simulink model "project5"  (R2021a)
settings: Solver=VariableStepAuto  StartTime=0.0  StopTime=350  RelTol=1e-3
undefined symbols (not defined in the file or in its folder): AXI4, Lite
libraries: hdlBasic x323, xbsIndex_r4 x1
(part 2 of 3)

== system project5/Subsystem1 ==
  sel_in : Inport
  theta_in : Inport  Port=2
  start : Inport  Port=3
  Data_in2 : Inport  Port=4
  Constant2 : hdlBasic/Constant  const=0  gui_display_data_type=Boolean  arith_type=Boolean  n_bits=16  bin_pt=14  preci_type=Single  exp_width=8  frac_width=24  explicit_period=off  period=1  XmcBlockStatus=1  maskContainerNames=tabcontainer1  block_type=constant  block_config=sysgen:Constant_config
  Constant6 : hdlBasic/Constant  const=0  gui_display_data_type=Fixed-point  arith_type=Signed (2's comp)  n_bits=20  bin_pt=10  preci_type=Single  exp_width=8  frac_width=24  explicit_period=off  period=1  XmcBlockStatus=1  maskContainerNames=tabcontainer1  block_type=constant  block_config=sysgen:Constant_config
  Delay : hdlBasic/Delay  rst=off  en=on  latency=1  reg_retiming=off  XmcBlockStatus=1  maskContainerNames=group1  block_type=delay  block_config=sysgen:Delay_config
  Delay1 : hdlBasic/Delay  rst=off  en=on  latency=1  reg_retiming=off  XmcBlockStatus=1  maskContainerNames=group1  block_type=delay  block_config=sysgen:Delay_config
  Delay2 : hdlBasic/Delay  rst=off  en=off  latency=2  reg_retiming=off  XmcBlockStatus=1  maskContainerNames=group1  block_type=delay  block_config=sysgen:Delay_config
  Delay3 : hdlBasic/Delay  rst=off  en=off  latency=1  reg_retiming=off  XmcBlockStatus=1  maskContainerNames=group1  block_type=delay  block_config=sysgen:Delay_config
  Delay4 : hdlBasic/Delay  rst=off  en=off  latency=1  reg_retiming=off  XmcBlockStatus=1  maskContainerNames=group1  block_type=delay  block_config=sysgen:Delay_config
  Mux : hdlBasic/Mux  inputs=2  en=off  latency=1  precision=Full  arith_type=Unsigned  n_bits=16  bin_pt=14  quantization=Truncate  overflow=Wrap  XmcBlockStatus=1  maskContainerNames=tabcontainer1  block_type=mux  block_config=sysgen:Mux_config
  Mux1 : hdlBasic/Mux  inputs=2  en=off  latency=1  precision=Full  arith_type=Unsigned  n_bits=16  bin_pt=14  quantization=Truncate  overflow=Wrap  XmcBlockStatus=1  maskContainerNames=tabcontainer1  block_type=mux  block_config=sysgen:Mux_config
  Vitis HLS : hdlBasic/Vitis HLS  anytable='C:\ELEC522\jg122\Project5_sinandcos\sincos\solution1'  fast_sim=off  display_datatype=off  rate_propagation_method=Simulink system period  model_file_path=''  latency=1  block_type=vitis_hls
      settings: infoedit=This block allows including C,C++ and SystemC source files in System Generator for DSP designs.
  Ctrl_out : Outport
  theta_out : Outport  Port=2
  result_out : Outport  Port=3
  y_out : Outport  Port=4
  wires:
  Vitis HLS/4 -> Delay/1
  Vitis HLS/5 -> Delay/2
  Delay1/1 -> y_out/1
  Vitis HLS/7 -> Delay1/2
  Vitis HLS/6 -> Delay1/1
  sel_in/1 -> Delay4/1, Mux/1, Mux1/1
  Delay/1 -> result_out/1, Mux/2
  Constant6/1 -> Mux1/3
  Data_in2/1 -> Mux1/2, Mux/3
  Mux1/1 -> Vitis HLS/4
  Mux/1 -> Delay2/1
  theta_in/1 -> Vitis HLS/3, Delay3/1
  Delay3/1 -> theta_out/1
  Delay2/1 -> Vitis HLS/5
  Delay4/1 -> Ctrl_out/1
  start/1 -> Vitis HLS/2
  Constant2/1 -> Vitis HLS/1

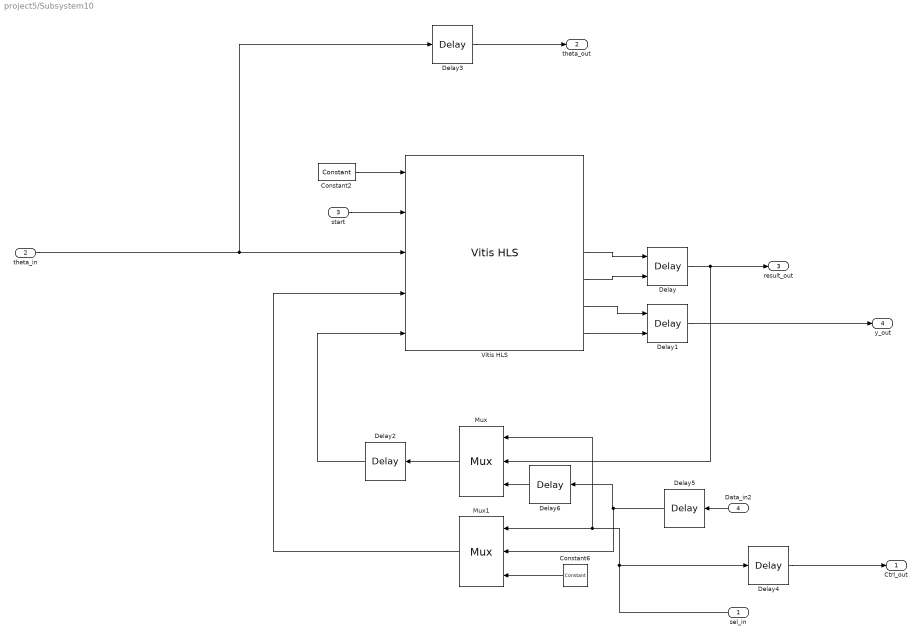
== system project5/Subsystem10 ==
  sel_in : Inport
  theta_in : Inport  Port=2
  start : Inport  Port=3
  Data_in2 : Inport  Port=4
  Constant2 : hdlBasic/Constant  const=0  gui_display_data_type=Boolean  arith_type=Boolean  n_bits=16  bin_pt=14  preci_type=Single  exp_width=8  frac_width=24  explicit_period=off  period=1  XmcBlockStatus=1  maskContainerNames=tabcontainer1  block_type=constant  block_config=sysgen:Constant_config
  Constant6 : hdlBasic/Constant  const=0  gui_display_data_type=Fixed-point  arith_type=Signed (2's comp)  n_bits=20  bin_pt=10  preci_type=Single  exp_width=8  frac_width=24  explicit_period=off  period=1  XmcBlockStatus=1  maskContainerNames=tabcontainer1  block_type=constant  block_config=sysgen:Constant_config
  Delay : hdlBasic/Delay  rst=off  en=on  latency=1  reg_retiming=off  XmcBlockStatus=1  maskContainerNames=group1  block_type=delay  block_config=sysgen:Delay_config
  Delay1 : hdlBasic/Delay  rst=off  en=on  latency=1  reg_retiming=off  XmcBlockStatus=1  maskContainerNames=group1  block_type=delay  block_config=sysgen:Delay_config
  Delay2 : hdlBasic/Delay  rst=off  en=off  latency=2  reg_retiming=off  XmcBlockStatus=1  maskContainerNames=group1  block_type=delay  block_config=sysgen:Delay_config
  Delay3 : hdlBasic/Delay  rst=off  en=off  latency=1  reg_retiming=off  XmcBlockStatus=1  maskContainerNames=group1  block_type=delay  block_config=sysgen:Delay_config
  Delay4 : hdlBasic/Delay  rst=off  en=off  latency=1  reg_retiming=off  XmcBlockStatus=1  maskContainerNames=group1  block_type=delay  block_config=sysgen:Delay_config
  Delay5 : hdlBasic/Delay  rst=off  en=off  latency=19  reg_retiming=off  XmcBlockStatus=1  maskContainerNames=group1  block_type=delay  block_config=sysgen:Delay_config
  Delay6 : hdlBasic/Delay  rst=off  en=off  latency=25  reg_retiming=off  XmcBlockStatus=1  maskContainerNames=group1  block_type=delay  block_config=sysgen:Delay_config
  Mux : hdlBasic/Mux  inputs=2  en=off  latency=1  precision=Full  arith_type=Unsigned  n_bits=16  bin_pt=14  quantization=Truncate  overflow=Wrap  XmcBlockStatus=1  maskContainerNames=tabcontainer1  block_type=mux  block_config=sysgen:Mux_config
  Mux1 : hdlBasic/Mux  inputs=2  en=off  latency=1  precision=Full  arith_type=Unsigned  n_bits=16  bin_pt=14  quantization=Truncate  overflow=Wrap  XmcBlockStatus=1  maskContainerNames=tabcontainer1  block_type=mux  block_config=sysgen:Mux_config
  Vitis HLS : hdlBasic/Vitis HLS  anytable='C:\ELEC522\jg122\Project5_sinandcos\sincos\solution1'  fast_sim=off  display_datatype=off  rate_propagation_method=Simulink system period  model_file_path=''  latency=1  block_type=vitis_hls
      settings: infoedit=This block allows including C,C++ and SystemC source files in System Generator for DSP designs.
  Ctrl_out : Outport
  theta_out : Outport  Port=2
  result_out : Outport  Port=3
  y_out : Outport  Port=4
  wires:
  Vitis HLS/4 -> Delay/1
  Vitis HLS/5 -> Delay/2
  Delay1/1 -> y_out/1
  Vitis HLS/7 -> Delay1/2
  Vitis HLS/6 -> Delay1/1
  Delay/1 -> result_out/1, Mux/2
  Constant6/1 -> Mux1/3
  Data_in2/1 -> Delay5/1
  Mux1/1 -> Vitis HLS/4
  Mux/1 -> Delay2/1
  theta_in/1 -> Vitis HLS/3, Delay3/1
  Delay3/1 -> theta_out/1
  Delay2/1 -> Vitis HLS/5
  Delay4/1 -> Ctrl_out/1
  Delay5/1 -> Mux1/2, Delay6/1
  Delay6/1 -> Mux/3
  sel_in/1 -> Mux/1, Mux1/1, Delay4/1
  start/1 -> Vitis HLS/2
  Constant2/1 -> Vitis HLS/1

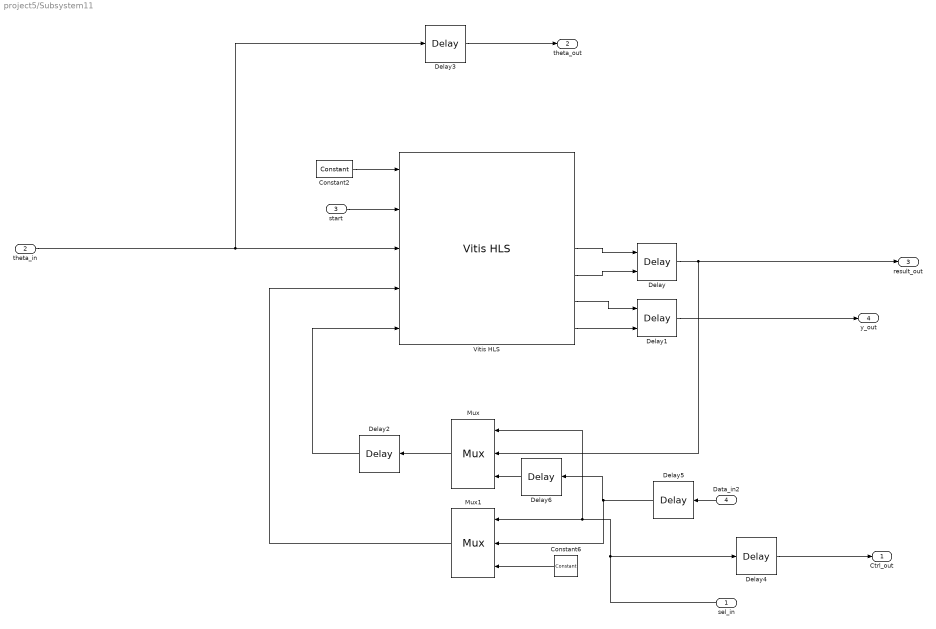
== system project5/Subsystem11 ==
  sel_in : Inport
  theta_in : Inport  Port=2
  start : Inport  Port=3
  Data_in2 : Inport  Port=4
  Constant2 : hdlBasic/Constant  const=0  gui_display_data_type=Boolean  arith_type=Boolean  n_bits=16  bin_pt=14  preci_type=Single  exp_width=8  frac_width=24  explicit_period=off  period=1  XmcBlockStatus=1  maskContainerNames=tabcontainer1  block_type=constant  block_config=sysgen:Constant_config
  Constant6 : hdlBasic/Constant  const=0  gui_display_data_type=Fixed-point  arith_type=Signed (2's comp)  n_bits=20  bin_pt=10  preci_type=Single  exp_width=8  frac_width=24  explicit_period=off  period=1  XmcBlockStatus=1  maskContainerNames=tabcontainer1  block_type=constant  block_config=sysgen:Constant_config
  Delay : hdlBasic/Delay  rst=off  en=on  latency=1  reg_retiming=off  XmcBlockStatus=1  maskContainerNames=group1  block_type=delay  block_config=sysgen:Delay_config
  Delay1 : hdlBasic/Delay  rst=off  en=on  latency=1  reg_retiming=off  XmcBlockStatus=1  maskContainerNames=group1  block_type=delay  block_config=sysgen:Delay_config
  Delay2 : hdlBasic/Delay  rst=off  en=off  latency=2  reg_retiming=off  XmcBlockStatus=1  maskContainerNames=group1  block_type=delay  block_config=sysgen:Delay_config
  Delay3 : hdlBasic/Delay  rst=off  en=off  latency=1  reg_retiming=off  XmcBlockStatus=1  maskContainerNames=group1  block_type=delay  block_config=sysgen:Delay_config
  Delay4 : hdlBasic/Delay  rst=off  en=off  latency=1  reg_retiming=off  XmcBlockStatus=1  maskContainerNames=group1  block_type=delay  block_config=sysgen:Delay_config
  Delay5 : hdlBasic/Delay  rst=off  en=off  latency=19  reg_retiming=off  XmcBlockStatus=1  maskContainerNames=group1  block_type=delay  block_config=sysgen:Delay_config
  Delay6 : hdlBasic/Delay  rst=off  en=off  latency=25  reg_retiming=off  XmcBlockStatus=1  maskContainerNames=group1  block_type=delay  block_config=sysgen:Delay_config
  Mux : hdlBasic/Mux  inputs=2  en=off  latency=1  precision=Full  arith_type=Unsigned  n_bits=16  bin_pt=14  quantization=Truncate  overflow=Wrap  XmcBlockStatus=1  maskContainerNames=tabcontainer1  block_type=mux  block_config=sysgen:Mux_config
  Mux1 : hdlBasic/Mux  inputs=2  en=off  latency=1  precision=Full  arith_type=Unsigned  n_bits=16  bin_pt=14  quantization=Truncate  overflow=Wrap  XmcBlockStatus=1  maskContainerNames=tabcontainer1  block_type=mux  block_config=sysgen:Mux_config
  Vitis HLS : hdlBasic/Vitis HLS  anytable='C:\ELEC522\jg122\Project5_sinandcos\sincos\solution1'  fast_sim=off  display_datatype=off  rate_propagation_method=Simulink system period  model_file_path=''  latency=1  block_type=vitis_hls
      settings: infoedit=This block allows including C,C++ and SystemC source files in System Generator for DSP designs.
  Ctrl_out : Outport
  theta_out : Outport  Port=2
  result_out : Outport  Port=3
  y_out : Outport  Port=4
  wires:
  Vitis HLS/4 -> Delay/1
  Vitis HLS/5 -> Delay/2
  Delay1/1 -> y_out/1
  Vitis HLS/7 -> Delay1/2
  Vitis HLS/6 -> Delay1/1
  Constant6/1 -> Mux1/3
  Data_in2/1 -> Delay5/1
  Mux1/1 -> Vitis HLS/4
  Mux/1 -> Delay2/1
  theta_in/1 -> Vitis HLS/3, Delay3/1
  Delay3/1 -> theta_out/1
  Delay2/1 -> Vitis HLS/5
  Delay4/1 -> Ctrl_out/1
  Delay5/1 -> Mux1/2, Delay6/1
  Delay6/1 -> Mux/3
  sel_in/1 -> Mux/1, Mux1/1, Delay4/1
  start/1 -> Vitis HLS/2
  Constant2/1 -> Vitis HLS/1
  Delay/1 -> result_out/1, Mux/2

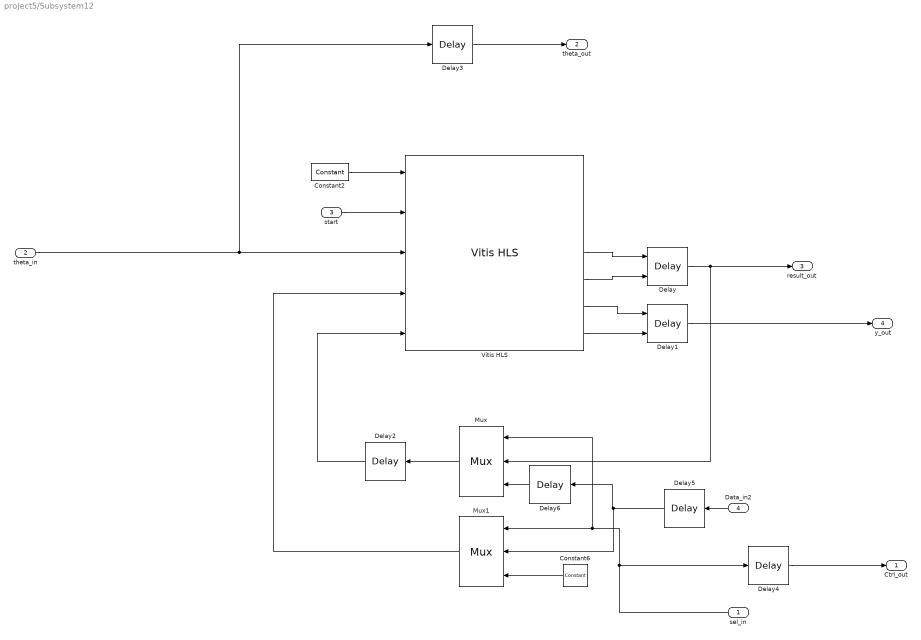
== system project5/Subsystem12 ==
  sel_in : Inport
  theta_in : Inport  Port=2
  start : Inport  Port=3
  Data_in2 : Inport  Port=4
  Constant2 : hdlBasic/Constant  const=0  gui_display_data_type=Boolean  arith_type=Boolean  n_bits=16  bin_pt=14  preci_type=Single  exp_width=8  frac_width=24  explicit_period=off  period=1  XmcBlockStatus=1  maskContainerNames=tabcontainer1  block_type=constant  block_config=sysgen:Constant_config
  Constant6 : hdlBasic/Constant  const=0  gui_display_data_type=Fixed-point  arith_type=Signed (2's comp)  n_bits=20  bin_pt=10  preci_type=Single  exp_width=8  frac_width=24  explicit_period=off  period=1  XmcBlockStatus=1  maskContainerNames=tabcontainer1  block_type=constant  block_config=sysgen:Constant_config
  Delay : hdlBasic/Delay  rst=off  en=on  latency=1  reg_retiming=off  XmcBlockStatus=1  maskContainerNames=group1  block_type=delay  block_config=sysgen:Delay_config
  Delay1 : hdlBasic/Delay  rst=off  en=on  latency=1  reg_retiming=off  XmcBlockStatus=1  maskContainerNames=group1  block_type=delay  block_config=sysgen:Delay_config
  Delay2 : hdlBasic/Delay  rst=off  en=off  latency=2  reg_retiming=off  XmcBlockStatus=1  maskContainerNames=group1  block_type=delay  block_config=sysgen:Delay_config
  Delay3 : hdlBasic/Delay  rst=off  en=off  latency=1  reg_retiming=off  XmcBlockStatus=1  maskContainerNames=group1  block_type=delay  block_config=sysgen:Delay_config
  Delay4 : hdlBasic/Delay  rst=off  en=off  latency=1  reg_retiming=off  XmcBlockStatus=1  maskContainerNames=group1  block_type=delay  block_config=sysgen:Delay_config
  Delay5 : hdlBasic/Delay  rst=off  en=off  latency=19  reg_retiming=off  XmcBlockStatus=1  maskContainerNames=group1  block_type=delay  block_config=sysgen:Delay_config
  Delay6 : hdlBasic/Delay  rst=off  en=off  latency=25  reg_retiming=off  XmcBlockStatus=1  maskContainerNames=group1  block_type=delay  block_config=sysgen:Delay_config
  Mux : hdlBasic/Mux  inputs=2  en=off  latency=1  precision=Full  arith_type=Unsigned  n_bits=16  bin_pt=14  quantization=Truncate  overflow=Wrap  XmcBlockStatus=1  maskContainerNames=tabcontainer1  block_type=mux  block_config=sysgen:Mux_config
  Mux1 : hdlBasic/Mux  inputs=2  en=off  latency=1  precision=Full  arith_type=Unsigned  n_bits=16  bin_pt=14  quantization=Truncate  overflow=Wrap  XmcBlockStatus=1  maskContainerNames=tabcontainer1  block_type=mux  block_config=sysgen:Mux_config
  Vitis HLS : hdlBasic/Vitis HLS  anytable='C:\ELEC522\jg122\Project5_sinandcos\sincos\solution1'  fast_sim=off  display_datatype=off  rate_propagation_method=Simulink system period  model_file_path=''  latency=1  block_type=vitis_hls
      settings: infoedit=This block allows including C,C++ and SystemC source files in System Generator for DSP designs.
  Ctrl_out : Outport
  theta_out : Outport  Port=2
  result_out : Outport  Port=3
  y_out : Outport  Port=4
  wires:
  Vitis HLS/4 -> Delay/1
  Vitis HLS/5 -> Delay/2
  Delay1/1 -> y_out/1
  Vitis HLS/7 -> Delay1/2
  Vitis HLS/6 -> Delay1/1
  Constant6/1 -> Mux1/3
  Data_in2/1 -> Delay5/1
  Mux1/1 -> Vitis HLS/4
  Mux/1 -> Delay2/1
  theta_in/1 -> Vitis HLS/3, Delay3/1
  Delay3/1 -> theta_out/1
  Delay2/1 -> Vitis HLS/5
  Delay4/1 -> Ctrl_out/1
  Delay5/1 -> Mux1/2, Delay6/1
  Delay6/1 -> Mux/3
  sel_in/1 -> Mux/1, Mux1/1, Delay4/1
  start/1 -> Vitis HLS/2
  Constant2/1 -> Vitis HLS/1
  Delay/1 -> result_out/1, Mux/2

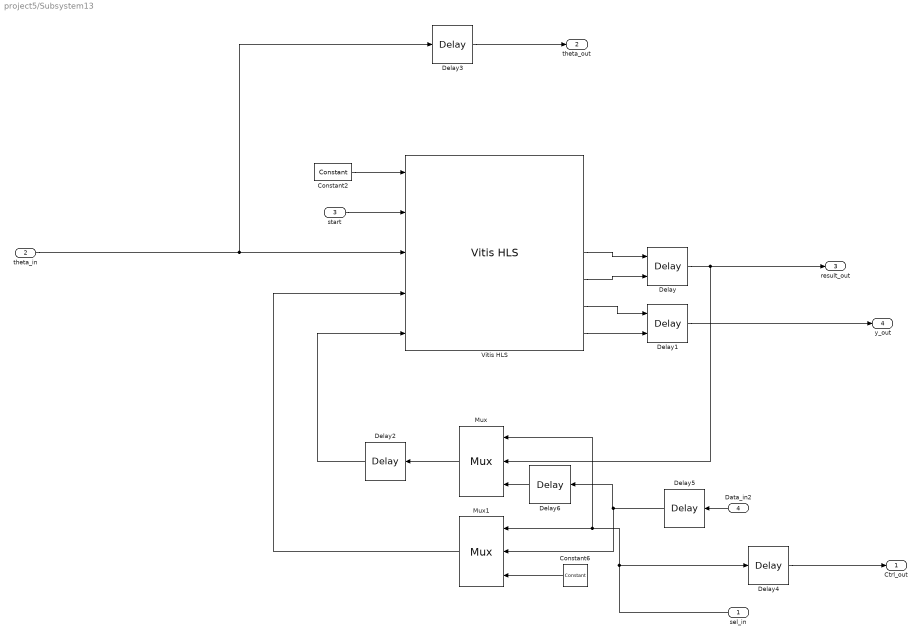
== system project5/Subsystem13 ==
  sel_in : Inport
  theta_in : Inport  Port=2
  start : Inport  Port=3
  Data_in2 : Inport  Port=4
  Constant2 : hdlBasic/Constant  const=0  gui_display_data_type=Boolean  arith_type=Boolean  n_bits=16  bin_pt=14  preci_type=Single  exp_width=8  frac_width=24  explicit_period=off  period=1  XmcBlockStatus=1  maskContainerNames=tabcontainer1  block_type=constant  block_config=sysgen:Constant_config
  Constant6 : hdlBasic/Constant  const=0  gui_display_data_type=Fixed-point  arith_type=Signed (2's comp)  n_bits=20  bin_pt=10  preci_type=Single  exp_width=8  frac_width=24  explicit_period=off  period=1  XmcBlockStatus=1  maskContainerNames=tabcontainer1  block_type=constant  block_config=sysgen:Constant_config
  Delay : hdlBasic/Delay  rst=off  en=on  latency=1  reg_retiming=off  XmcBlockStatus=1  maskContainerNames=group1  block_type=delay  block_config=sysgen:Delay_config
  Delay1 : hdlBasic/Delay  rst=off  en=on  latency=1  reg_retiming=off  XmcBlockStatus=1  maskContainerNames=group1  block_type=delay  block_config=sysgen:Delay_config
  Delay2 : hdlBasic/Delay  rst=off  en=off  latency=2  reg_retiming=off  XmcBlockStatus=1  maskContainerNames=group1  block_type=delay  block_config=sysgen:Delay_config
  Delay3 : hdlBasic/Delay  rst=off  en=off  latency=1  reg_retiming=off  XmcBlockStatus=1  maskContainerNames=group1  block_type=delay  block_config=sysgen:Delay_config
  Delay4 : hdlBasic/Delay  rst=off  en=off  latency=1  reg_retiming=off  XmcBlockStatus=1  maskContainerNames=group1  block_type=delay  block_config=sysgen:Delay_config
  Delay5 : hdlBasic/Delay  rst=off  en=off  latency=19  reg_retiming=off  XmcBlockStatus=1  maskContainerNames=group1  block_type=delay  block_config=sysgen:Delay_config
  Delay6 : hdlBasic/Delay  rst=off  en=off  latency=25  reg_retiming=off  XmcBlockStatus=1  maskContainerNames=group1  block_type=delay  block_config=sysgen:Delay_config
  Mux : hdlBasic/Mux  inputs=2  en=off  latency=1  precision=Full  arith_type=Unsigned  n_bits=16  bin_pt=14  quantization=Truncate  overflow=Wrap  XmcBlockStatus=1  maskContainerNames=tabcontainer1  block_type=mux  block_config=sysgen:Mux_config
  Mux1 : hdlBasic/Mux  inputs=2  en=off  latency=1  precision=Full  arith_type=Unsigned  n_bits=16  bin_pt=14  quantization=Truncate  overflow=Wrap  XmcBlockStatus=1  maskContainerNames=tabcontainer1  block_type=mux  block_config=sysgen:Mux_config
  Vitis HLS : hdlBasic/Vitis HLS  anytable='C:\ELEC522\jg122\Project5_sinandcos\sincos\solution1'  fast_sim=off  display_datatype=off  rate_propagation_method=Simulink system period  model_file_path=''  latency=1  block_type=vitis_hls
      settings: infoedit=This block allows including C,C++ and SystemC source files in System Generator for DSP designs.
  Ctrl_out : Outport
  theta_out : Outport  Port=2
  result_out : Outport  Port=3
  y_out : Outport  Port=4
  wires:
  Vitis HLS/4 -> Delay/1
  Vitis HLS/5 -> Delay/2
  Delay1/1 -> y_out/1
  Vitis HLS/7 -> Delay1/2
  Vitis HLS/6 -> Delay1/1
  Constant6/1 -> Mux1/3
  Data_in2/1 -> Delay5/1
  Mux1/1 -> Vitis HLS/4
  Mux/1 -> Delay2/1
  theta_in/1 -> Vitis HLS/3, Delay3/1
  Delay3/1 -> theta_out/1
  Delay2/1 -> Vitis HLS/5
  Delay4/1 -> Ctrl_out/1
  Delay5/1 -> Mux1/2, Delay6/1
  Delay6/1 -> Mux/3
  sel_in/1 -> Mux/1, Mux1/1, Delay4/1
  start/1 -> Vitis HLS/2
  Constant2/1 -> Vitis HLS/1
  Delay/1 -> result_out/1, Mux/2

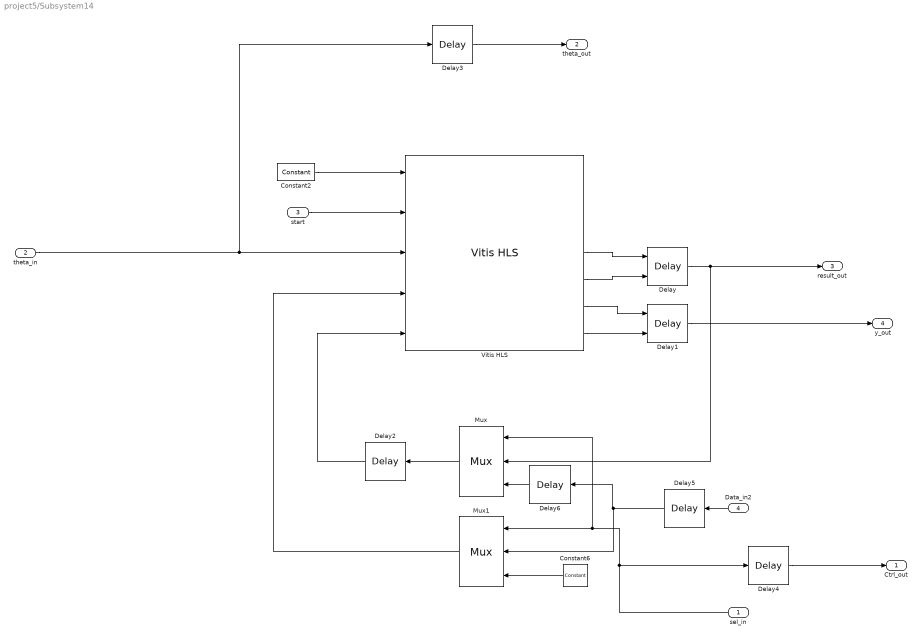
== system project5/Subsystem14 ==
  sel_in : Inport
  theta_in : Inport  Port=2
  start : Inport  Port=3
  Data_in2 : Inport  Port=4
  Constant2 : hdlBasic/Constant  const=0  gui_display_data_type=Boolean  arith_type=Boolean  n_bits=16  bin_pt=14  preci_type=Single  exp_width=8  frac_width=24  explicit_period=off  period=1  XmcBlockStatus=1  maskContainerNames=tabcontainer1  block_type=constant  block_config=sysgen:Constant_config
  Constant6 : hdlBasic/Constant  const=0  gui_display_data_type=Fixed-point  arith_type=Signed (2's comp)  n_bits=20  bin_pt=10  preci_type=Single  exp_width=8  frac_width=24  explicit_period=off  period=1  XmcBlockStatus=1  maskContainerNames=tabcontainer1  block_type=constant  block_config=sysgen:Constant_config
  Delay : hdlBasic/Delay  rst=off  en=on  latency=1  reg_retiming=off  XmcBlockStatus=1  maskContainerNames=group1  block_type=delay  block_config=sysgen:Delay_config
  Delay1 : hdlBasic/Delay  rst=off  en=on  latency=1  reg_retiming=off  XmcBlockStatus=1  maskContainerNames=group1  block_type=delay  block_config=sysgen:Delay_config
  Delay2 : hdlBasic/Delay  rst=off  en=off  latency=2  reg_retiming=off  XmcBlockStatus=1  maskContainerNames=group1  block_type=delay  block_config=sysgen:Delay_config
  Delay3 : hdlBasic/Delay  rst=off  en=off  latency=1  reg_retiming=off  XmcBlockStatus=1  maskContainerNames=group1  block_type=delay  block_config=sysgen:Delay_config
  Delay4 : hdlBasic/Delay  rst=off  en=off  latency=1  reg_retiming=off  XmcBlockStatus=1  maskContainerNames=group1  block_type=delay  block_config=sysgen:Delay_config
  Delay5 : hdlBasic/Delay  rst=off  en=off  latency=19  reg_retiming=off  XmcBlockStatus=1  maskContainerNames=group1  block_type=delay  block_config=sysgen:Delay_config
  Delay6 : hdlBasic/Delay  rst=off  en=off  latency=25  reg_retiming=off  XmcBlockStatus=1  maskContainerNames=group1  block_type=delay  block_config=sysgen:Delay_config
  Mux : hdlBasic/Mux  inputs=2  en=off  latency=1  precision=Full  arith_type=Unsigned  n_bits=16  bin_pt=14  quantization=Truncate  overflow=Wrap  XmcBlockStatus=1  maskContainerNames=tabcontainer1  block_type=mux  block_config=sysgen:Mux_config
  Mux1 : hdlBasic/Mux  inputs=2  en=off  latency=1  precision=Full  arith_type=Unsigned  n_bits=16  bin_pt=14  quantization=Truncate  overflow=Wrap  XmcBlockStatus=1  maskContainerNames=tabcontainer1  block_type=mux  block_config=sysgen:Mux_config
  Vitis HLS : hdlBasic/Vitis HLS  anytable='C:\ELEC522\jg122\Project5_sinandcos\sincos\solution1'  fast_sim=off  display_datatype=off  rate_propagation_method=Simulink system period  model_file_path=''  latency=1  block_type=vitis_hls
      settings: infoedit=This block allows including C,C++ and SystemC source files in System Generator for DSP designs.
  Ctrl_out : Outport
  theta_out : Outport  Port=2
  result_out : Outport  Port=3
  y_out : Outport  Port=4
  wires:
  Vitis HLS/4 -> Delay/1
  Vitis HLS/5 -> Delay/2
  Delay1/1 -> y_out/1
  Vitis HLS/7 -> Delay1/2
  Vitis HLS/6 -> Delay1/1
  Constant6/1 -> Mux1/3
  Data_in2/1 -> Delay5/1
  Mux1/1 -> Vitis HLS/4
  Mux/1 -> Delay2/1
  theta_in/1 -> Vitis HLS/3, Delay3/1
  Delay3/1 -> theta_out/1
  Delay2/1 -> Vitis HLS/5
  Delay4/1 -> Ctrl_out/1
  Delay5/1 -> Mux1/2, Delay6/1
  Delay6/1 -> Mux/3
  sel_in/1 -> Mux/1, Mux1/1, Delay4/1
  start/1 -> Vitis HLS/2
  Constant2/1 -> Vitis HLS/1
  Delay/1 -> result_out/1, Mux/2

== system project5/Subsystem15 ==
  SIgnal_ctrl : Inport
  Signal_input1 : Inport  Port=2
  start : Inport  Port=3
  Constant1 : hdlBasic/Constant  const=0  gui_display_data_type=Boolean  arith_type=Boolean  n_bits=16  bin_pt=14  preci_type=Single  exp_width=8  frac_width=24  explicit_period=off  period=1  XmcBlockStatus=1  maskContainerNames=tabcontainer1  block_type=constant  block_config=sysgen:Constant_config
  Constant3 : hdlBasic/Constant  const=0  gui_display_data_type=Fixed-point  arith_type=Signed (2's comp)  n_bits=20  bin_pt=10  preci_type=Single  exp_width=8  frac_width=24  explicit_period=off  period=1  XmcBlockStatus=1  maskContainerNames=tabcontainer1  block_type=constant  block_config=sysgen:Constant_config
  Delay1 : hdlBasic/Delay  rst=off  en=off  latency=5  reg_retiming=off  XmcBlockStatus=1  maskContainerNames=group1  block_type=delay  block_config=sysgen:Delay_config
  Delay2 : hdlBasic/Delay  rst=off  en=off  latency=2  reg_retiming=off  XmcBlockStatus=1  maskContainerNames=group1  block_type=delay  block_config=sysgen:Delay_config
  Delay3 : hdlBasic/Delay  rst=off  en=off  latency=20  reg_retiming=off  XmcBlockStatus=1  maskContainerNames=group1  block_type=delay  block_config=sysgen:Delay_config
  Delay4 : hdlBasic/Delay  rst=off  en=on  latency=1  reg_retiming=off  XmcBlockStatus=1  maskContainerNames=group1  block_type=delay  block_config=sysgen:Delay_config
  Delay5 : hdlBasic/Delay  rst=off  en=on  latency=1  reg_retiming=off  XmcBlockStatus=1  maskContainerNames=group1  block_type=delay  block_config=sysgen:Delay_config
  Delay6 : hdlBasic/Delay  rst=off  en=off  latency=25  reg_retiming=off  XmcBlockStatus=1  maskContainerNames=group1  block_type=delay  block_config=sysgen:Delay_config
  Delay7 : hdlBasic/Delay  rst=off  en=off  latency=79  reg_retiming=off  XmcBlockStatus=1  maskContainerNames=group1  block_type=delay  block_config=sysgen:Delay_config
  Delay8 : hdlBasic/Delay  rst=off  en=off  latency=23  reg_retiming=off  XmcBlockStatus=1  maskContainerNames=group1  block_type=delay  block_config=sysgen:Delay_config
  Mux : hdlBasic/Mux  inputs=2  en=off  latency=1  precision=Full  arith_type=Unsigned  n_bits=16  bin_pt=14  quantization=Truncate  overflow=Wrap  XmcBlockStatus=1  maskContainerNames=tabcontainer1  block_type=mux  block_config=sysgen:Mux_config
  Mux1 : hdlBasic/Mux  inputs=2  en=off  latency=1  precision=Full  arith_type=Unsigned  n_bits=16  bin_pt=14  quantization=Truncate  overflow=Wrap  XmcBlockStatus=1  maskContainerNames=tabcontainer1  block_type=mux  block_config=sysgen:Mux_config
  Vitis HLS : hdlBasic/Vitis HLS  anytable='C:\ELEC522\jg122\Project5_atan\atan\solution1'  fast_sim=off  display_datatype=on  rate_propagation_method=Simulink system period  model_file_path=''  latency=1  block_type=vitis_hls
      settings: infoedit=This block allows including C,C++ and SystemC source files in System Generator for DSP designs.
  Ctrl_out : Outport
  atan_out1 : Outport  Port=2
  R_out : Outport  Port=3
  wires:
  Vitis HLS/4 -> Delay4/1
  Vitis HLS/6 -> Delay5/1, Delay1/1
  SIgnal_ctrl/1 -> Delay7/1
  Constant3/1 -> Mux1/3
  Mux/1 -> Delay2/1
  Vitis HLS/5 -> Delay4/2
  Vitis HLS/7 -> Delay5/2
  Delay4/1 -> atan_out1/1
  Delay2/1 -> Vitis HLS/3
  Mux1/1 -> Vitis HLS/4
  Delay5/1 -> Delay8/1
  Delay3/1 -> Ctrl_out/1
  Delay1/1 -> Mux/2
  Delay7/1 -> Mux1/1, Delay3/1, Mux/1
  Signal_input1/1 -> Delay6/1, Mux1/2
  Delay6/1 -> Mux/3
  Delay8/1 -> R_out/1
  start/1 -> Vitis HLS/2
  Constant1/1 -> Vitis HLS/1

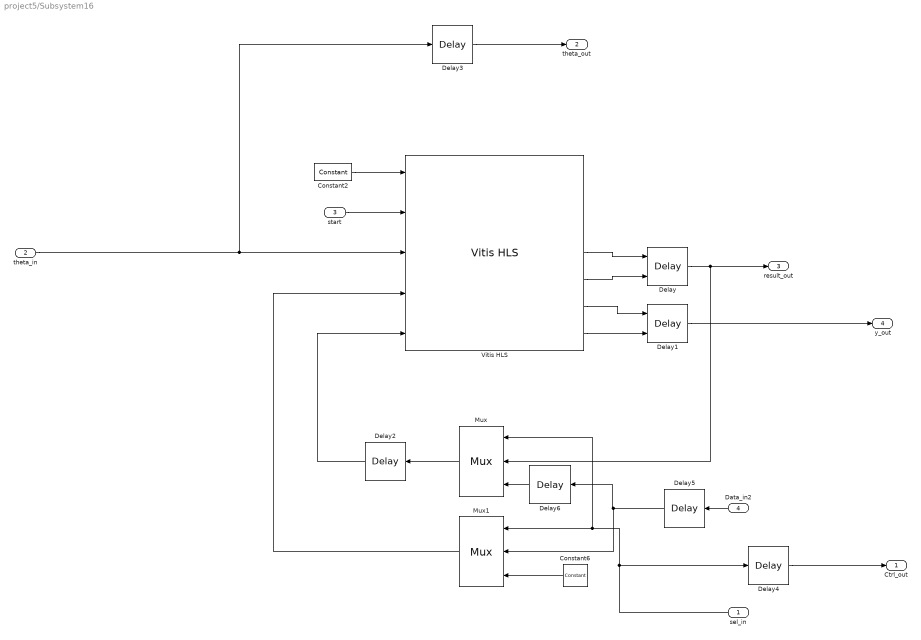
== system project5/Subsystem16 ==
  sel_in : Inport
  theta_in : Inport  Port=2
  start : Inport  Port=3
  Data_in2 : Inport  Port=4
  Constant2 : hdlBasic/Constant  const=0  gui_display_data_type=Boolean  arith_type=Boolean  n_bits=16  bin_pt=14  preci_type=Single  exp_width=8  frac_width=24  explicit_period=off  period=1  XmcBlockStatus=1  maskContainerNames=tabcontainer1  block_type=constant  block_config=sysgen:Constant_config
  Constant6 : hdlBasic/Constant  const=0  gui_display_data_type=Fixed-point  arith_type=Signed (2's comp)  n_bits=20  bin_pt=10  preci_type=Single  exp_width=8  frac_width=24  explicit_period=off  period=1  XmcBlockStatus=1  maskContainerNames=tabcontainer1  block_type=constant  block_config=sysgen:Constant_config
  Delay : hdlBasic/Delay  rst=off  en=on  latency=1  reg_retiming=off  XmcBlockStatus=1  maskContainerNames=group1  block_type=delay  block_config=sysgen:Delay_config
  Delay1 : hdlBasic/Delay  rst=off  en=on  latency=1  reg_retiming=off  XmcBlockStatus=1  maskContainerNames=group1  block_type=delay  block_config=sysgen:Delay_config
  Delay2 : hdlBasic/Delay  rst=off  en=off  latency=2  reg_retiming=off  XmcBlockStatus=1  maskContainerNames=group1  block_type=delay  block_config=sysgen:Delay_config
  Delay3 : hdlBasic/Delay  rst=off  en=off  latency=1  reg_retiming=off  XmcBlockStatus=1  maskContainerNames=group1  block_type=delay  block_config=sysgen:Delay_config
  Delay4 : hdlBasic/Delay  rst=off  en=off  latency=1  reg_retiming=off  XmcBlockStatus=1  maskContainerNames=group1  block_type=delay  block_config=sysgen:Delay_config
  Delay5 : hdlBasic/Delay  rst=off  en=off  latency=19  reg_retiming=off  XmcBlockStatus=1  maskContainerNames=group1  block_type=delay  block_config=sysgen:Delay_config
  Delay6 : hdlBasic/Delay  rst=off  en=off  latency=25  reg_retiming=off  XmcBlockStatus=1  maskContainerNames=group1  block_type=delay  block_config=sysgen:Delay_config
  Mux : hdlBasic/Mux  inputs=2  en=off  latency=1  precision=Full  arith_type=Unsigned  n_bits=16  bin_pt=14  quantization=Truncate  overflow=Wrap  XmcBlockStatus=1  maskContainerNames=tabcontainer1  block_type=mux  block_config=sysgen:Mux_config
  Mux1 : hdlBasic/Mux  inputs=2  en=off  latency=1  precision=Full  arith_type=Unsigned  n_bits=16  bin_pt=14  quantization=Truncate  overflow=Wrap  XmcBlockStatus=1  maskContainerNames=tabcontainer1  block_type=mux  block_config=sysgen:Mux_config
  Vitis HLS : hdlBasic/Vitis HLS  anytable='C:\ELEC522\jg122\Project5_sinandcos\sincos\solution1'  fast_sim=off  display_datatype=off  rate_propagation_method=Simulink system period  model_file_path=''  latency=1  block_type=vitis_hls
      settings: infoedit=This block allows including C,C++ and SystemC source files in System Generator for DSP designs.
  Ctrl_out : Outport
  theta_out : Outport  Port=2
  result_out : Outport  Port=3
  y_out : Outport  Port=4
  wires:
  Vitis HLS/4 -> Delay/1
  Vitis HLS/5 -> Delay/2
  Delay1/1 -> y_out/1
  Vitis HLS/7 -> Delay1/2
  Vitis HLS/6 -> Delay1/1
  Delay/1 -> result_out/1, Mux/2
  Constant6/1 -> Mux1/3
  Data_in2/1 -> Delay5/1
  Mux1/1 -> Vitis HLS/4
  Mux/1 -> Delay2/1
  theta_in/1 -> Vitis HLS/3, Delay3/1
  Delay3/1 -> theta_out/1
  Delay2/1 -> Vitis HLS/5
  Delay4/1 -> Ctrl_out/1
  Delay5/1 -> Mux1/2, Delay6/1
  Delay6/1 -> Mux/3
  sel_in/1 -> Mux/1, Mux1/1, Delay4/1
  start/1 -> Vitis HLS/2
  Constant2/1 -> Vitis HLS/1

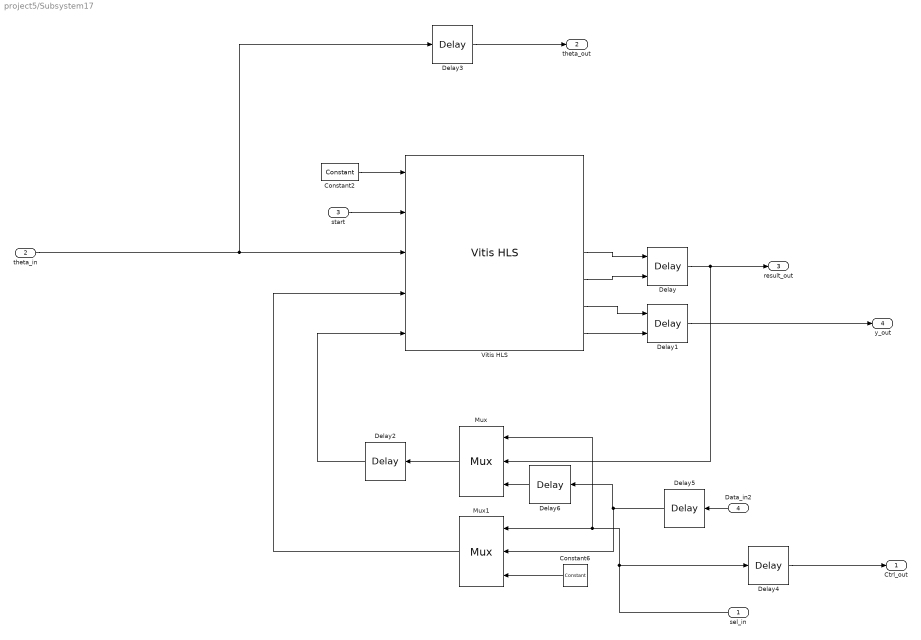
== system project5/Subsystem17 ==
  sel_in : Inport
  theta_in : Inport  Port=2
  start : Inport  Port=3
  Data_in2 : Inport  Port=4
  Constant2 : hdlBasic/Constant  const=0  gui_display_data_type=Boolean  arith_type=Boolean  n_bits=16  bin_pt=14  preci_type=Single  exp_width=8  frac_width=24  explicit_period=off  period=1  XmcBlockStatus=1  maskContainerNames=tabcontainer1  block_type=constant  block_config=sysgen:Constant_config
  Constant6 : hdlBasic/Constant  const=0  gui_display_data_type=Fixed-point  arith_type=Signed (2's comp)  n_bits=20  bin_pt=10  preci_type=Single  exp_width=8  frac_width=24  explicit_period=off  period=1  XmcBlockStatus=1  maskContainerNames=tabcontainer1  block_type=constant  block_config=sysgen:Constant_config
  Delay : hdlBasic/Delay  rst=off  en=on  latency=1  reg_retiming=off  XmcBlockStatus=1  maskContainerNames=group1  block_type=delay  block_config=sysgen:Delay_config
  Delay1 : hdlBasic/Delay  rst=off  en=on  latency=1  reg_retiming=off  XmcBlockStatus=1  maskContainerNames=group1  block_type=delay  block_config=sysgen:Delay_config
  Delay2 : hdlBasic/Delay  rst=off  en=off  latency=2  reg_retiming=off  XmcBlockStatus=1  maskContainerNames=group1  block_type=delay  block_config=sysgen:Delay_config
  Delay3 : hdlBasic/Delay  rst=off  en=off  latency=1  reg_retiming=off  XmcBlockStatus=1  maskContainerNames=group1  block_type=delay  block_config=sysgen:Delay_config
  Delay4 : hdlBasic/Delay  rst=off  en=off  latency=1  reg_retiming=off  XmcBlockStatus=1  maskContainerNames=group1  block_type=delay  block_config=sysgen:Delay_config
  Delay5 : hdlBasic/Delay  rst=off  en=off  latency=19  reg_retiming=off  XmcBlockStatus=1  maskContainerNames=group1  block_type=delay  block_config=sysgen:Delay_config
  Delay6 : hdlBasic/Delay  rst=off  en=off  latency=25  reg_retiming=off  XmcBlockStatus=1  maskContainerNames=group1  block_type=delay  block_config=sysgen:Delay_config
  Mux : hdlBasic/Mux  inputs=2  en=off  latency=1  precision=Full  arith_type=Unsigned  n_bits=16  bin_pt=14  quantization=Truncate  overflow=Wrap  XmcBlockStatus=1  maskContainerNames=tabcontainer1  block_type=mux  block_config=sysgen:Mux_config
  Mux1 : hdlBasic/Mux  inputs=2  en=off  latency=1  precision=Full  arith_type=Unsigned  n_bits=16  bin_pt=14  quantization=Truncate  overflow=Wrap  XmcBlockStatus=1  maskContainerNames=tabcontainer1  block_type=mux  block_config=sysgen:Mux_config
  Vitis HLS : hdlBasic/Vitis HLS  anytable='C:\ELEC522\jg122\Project5_sinandcos\sincos\solution1'  fast_sim=off  display_datatype=off  rate_propagation_method=Simulink system period  model_file_path=''  latency=1  block_type=vitis_hls
      settings: infoedit=This block allows including C,C++ and SystemC source files in System Generator for DSP designs.
  Ctrl_out : Outport
  theta_out : Outport  Port=2
  result_out : Outport  Port=3
  y_out : Outport  Port=4
  wires:
  Vitis HLS/4 -> Delay/1
  Vitis HLS/5 -> Delay/2
  Delay1/1 -> y_out/1
  Vitis HLS/7 -> Delay1/2
  Vitis HLS/6 -> Delay1/1
  Delay/1 -> result_out/1, Mux/2
  Constant6/1 -> Mux1/3
  Data_in2/1 -> Delay5/1
  Mux1/1 -> Vitis HLS/4
  Mux/1 -> Delay2/1
  theta_in/1 -> Vitis HLS/3, Delay3/1
  Delay3/1 -> theta_out/1
  Delay2/1 -> Vitis HLS/5
  Delay4/1 -> Ctrl_out/1
  Delay5/1 -> Mux1/2, Delay6/1
  Delay6/1 -> Mux/3
  sel_in/1 -> Mux/1, Mux1/1, Delay4/1
  Constant2/1 -> Vitis HLS/1
  start/1 -> Vitis HLS/2

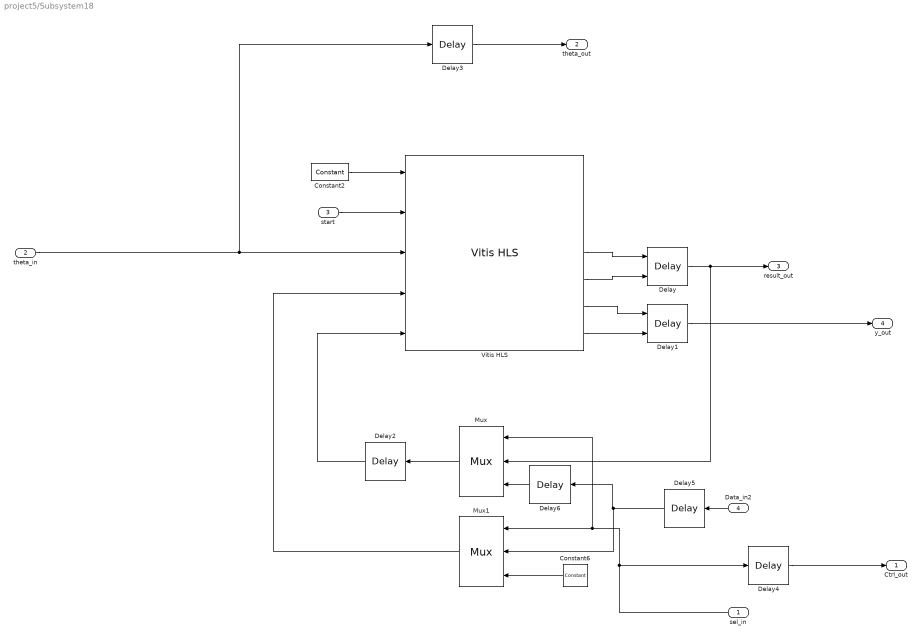
== system project5/Subsystem18 ==
  sel_in : Inport
  theta_in : Inport  Port=2
  start : Inport  Port=3
  Data_in2 : Inport  Port=4
  Constant2 : hdlBasic/Constant  const=0  gui_display_data_type=Boolean  arith_type=Boolean  n_bits=16  bin_pt=14  preci_type=Single  exp_width=8  frac_width=24  explicit_period=off  period=1  XmcBlockStatus=1  maskContainerNames=tabcontainer1  block_type=constant  block_config=sysgen:Constant_config
  Constant6 : hdlBasic/Constant  const=0  gui_display_data_type=Fixed-point  arith_type=Signed (2's comp)  n_bits=20  bin_pt=10  preci_type=Single  exp_width=8  frac_width=24  explicit_period=off  period=1  XmcBlockStatus=1  maskContainerNames=tabcontainer1  block_type=constant  block_config=sysgen:Constant_config
  Delay : hdlBasic/Delay  rst=off  en=on  latency=1  reg_retiming=off  XmcBlockStatus=1  maskContainerNames=group1  block_type=delay  block_config=sysgen:Delay_config
  Delay1 : hdlBasic/Delay  rst=off  en=on  latency=1  reg_retiming=off  XmcBlockStatus=1  maskContainerNames=group1  block_type=delay  block_config=sysgen:Delay_config
  Delay2 : hdlBasic/Delay  rst=off  en=off  latency=2  reg_retiming=off  XmcBlockStatus=1  maskContainerNames=group1  block_type=delay  block_config=sysgen:Delay_config
  Delay3 : hdlBasic/Delay  rst=off  en=off  latency=1  reg_retiming=off  XmcBlockStatus=1  maskContainerNames=group1  block_type=delay  block_config=sysgen:Delay_config
  Delay4 : hdlBasic/Delay  rst=off  en=off  latency=1  reg_retiming=off  XmcBlockStatus=1  maskContainerNames=group1  block_type=delay  block_config=sysgen:Delay_config
  Delay5 : hdlBasic/Delay  rst=off  en=off  latency=19  reg_retiming=off  XmcBlockStatus=1  maskContainerNames=group1  block_type=delay  block_config=sysgen:Delay_config
  Delay6 : hdlBasic/Delay  rst=off  en=off  latency=25  reg_retiming=off  XmcBlockStatus=1  maskContainerNames=group1  block_type=delay  block_config=sysgen:Delay_config
  Mux : hdlBasic/Mux  inputs=2  en=off  latency=1  precision=Full  arith_type=Unsigned  n_bits=16  bin_pt=14  quantization=Truncate  overflow=Wrap  XmcBlockStatus=1  maskContainerNames=tabcontainer1  block_type=mux  block_config=sysgen:Mux_config
  Mux1 : hdlBasic/Mux  inputs=2  en=off  latency=1  precision=Full  arith_type=Unsigned  n_bits=16  bin_pt=14  quantization=Truncate  overflow=Wrap  XmcBlockStatus=1  maskContainerNames=tabcontainer1  block_type=mux  block_config=sysgen:Mux_config
  Vitis HLS : hdlBasic/Vitis HLS  anytable='C:\ELEC522\jg122\Project5_sinandcos\sincos\solution1'  fast_sim=off  display_datatype=off  rate_propagation_method=Simulink system period  model_file_path=''  latency=1  block_type=vitis_hls
      settings: infoedit=This block allows including C,C++ and SystemC source files in System Generator for DSP designs.
  Ctrl_out : Outport
  theta_out : Outport  Port=2
  result_out : Outport  Port=3
  y_out : Outport  Port=4
  wires:
  Vitis HLS/4 -> Delay/1
  Vitis HLS/5 -> Delay/2
  Delay1/1 -> y_out/1
  Vitis HLS/7 -> Delay1/2
  Vitis HLS/6 -> Delay1/1
  Delay/1 -> result_out/1, Mux/2
  Constant6/1 -> Mux1/3
  Data_in2/1 -> Delay5/1
  Mux1/1 -> Vitis HLS/4
  Mux/1 -> Delay2/1
  theta_in/1 -> Vitis HLS/3, Delay3/1
  Delay3/1 -> theta_out/1
  Delay2/1 -> Vitis HLS/5
  Delay4/1 -> Ctrl_out/1
  Delay5/1 -> Mux1/2, Delay6/1
  Delay6/1 -> Mux/3
  sel_in/1 -> Mux/1, Mux1/1, Delay4/1
  Constant2/1 -> Vitis HLS/1
  start/1 -> Vitis HLS/2

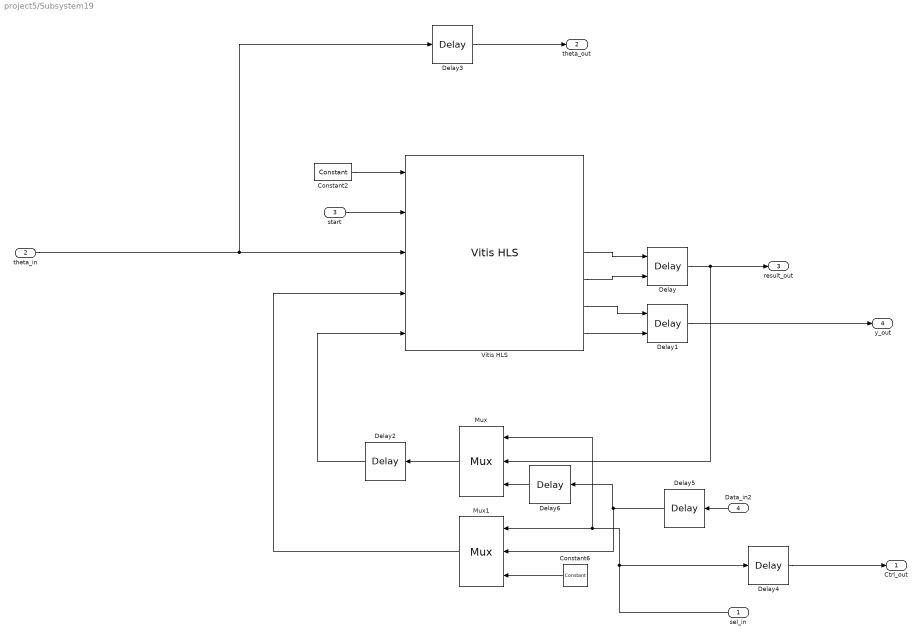
== system project5/Subsystem19 ==
  sel_in : Inport
  theta_in : Inport  Port=2
  start : Inport  Port=3
  Data_in2 : Inport  Port=4
  Constant2 : hdlBasic/Constant  const=0  gui_display_data_type=Boolean  arith_type=Boolean  n_bits=16  bin_pt=14  preci_type=Single  exp_width=8  frac_width=24  explicit_period=off  period=1  XmcBlockStatus=1  maskContainerNames=tabcontainer1  block_type=constant  block_config=sysgen:Constant_config
  Constant6 : hdlBasic/Constant  const=0  gui_display_data_type=Fixed-point  arith_type=Signed (2's comp)  n_bits=20  bin_pt=10  preci_type=Single  exp_width=8  frac_width=24  explicit_period=off  period=1  XmcBlockStatus=1  maskContainerNames=tabcontainer1  block_type=constant  block_config=sysgen:Constant_config
  Delay : hdlBasic/Delay  rst=off  en=on  latency=1  reg_retiming=off  XmcBlockStatus=1  maskContainerNames=group1  block_type=delay  block_config=sysgen:Delay_config
  Delay1 : hdlBasic/Delay  rst=off  en=on  latency=1  reg_retiming=off  XmcBlockStatus=1  maskContainerNames=group1  block_type=delay  block_config=sysgen:Delay_config
  Delay2 : hdlBasic/Delay  rst=off  en=off  latency=2  reg_retiming=off  XmcBlockStatus=1  maskContainerNames=group1  block_type=delay  block_config=sysgen:Delay_config
  Delay3 : hdlBasic/Delay  rst=off  en=off  latency=1  reg_retiming=off  XmcBlockStatus=1  maskContainerNames=group1  block_type=delay  block_config=sysgen:Delay_config
  Delay4 : hdlBasic/Delay  rst=off  en=off  latency=1  reg_retiming=off  XmcBlockStatus=1  maskContainerNames=group1  block_type=delay  block_config=sysgen:Delay_config
  Delay5 : hdlBasic/Delay  rst=off  en=off  latency=19  reg_retiming=off  XmcBlockStatus=1  maskContainerNames=group1  block_type=delay  block_config=sysgen:Delay_config
  Delay6 : hdlBasic/Delay  rst=off  en=off  latency=25  reg_retiming=off  XmcBlockStatus=1  maskContainerNames=group1  block_type=delay  block_config=sysgen:Delay_config
  Mux : hdlBasic/Mux  inputs=2  en=off  latency=1  precision=Full  arith_type=Unsigned  n_bits=16  bin_pt=14  quantization=Truncate  overflow=Wrap  XmcBlockStatus=1  maskContainerNames=tabcontainer1  block_type=mux  block_config=sysgen:Mux_config
  Mux1 : hdlBasic/Mux  inputs=2  en=off  latency=1  precision=Full  arith_type=Unsigned  n_bits=16  bin_pt=14  quantization=Truncate  overflow=Wrap  XmcBlockStatus=1  maskContainerNames=tabcontainer1  block_type=mux  block_config=sysgen:Mux_config
  Vitis HLS : hdlBasic/Vitis HLS  anytable='C:\ELEC522\jg122\Project5_sinandcos\sincos\solution1'  fast_sim=off  display_datatype=off  rate_propagation_method=Simulink system period  model_file_path=''  latency=1  block_type=vitis_hls
      settings: infoedit=This block allows including C,C++ and SystemC source files in System Generator for DSP designs.
  Ctrl_out : Outport
  theta_out : Outport  Port=2
  result_out : Outport  Port=3
  y_out : Outport  Port=4
  wires:
  Vitis HLS/4 -> Delay/1
  Vitis HLS/5 -> Delay/2
  Delay1/1 -> y_out/1
  Vitis HLS/7 -> Delay1/2
  Vitis HLS/6 -> Delay1/1
  Delay/1 -> result_out/1, Mux/2
  Constant6/1 -> Mux1/3
  Data_in2/1 -> Delay5/1
  Mux1/1 -> Vitis HLS/4
  Mux/1 -> Delay2/1
  theta_in/1 -> Vitis HLS/3, Delay3/1
  Delay3/1 -> theta_out/1
  Delay2/1 -> Vitis HLS/5
  Delay4/1 -> Ctrl_out/1
  Delay5/1 -> Mux1/2, Delay6/1
  Delay6/1 -> Mux/3
  sel_in/1 -> Mux/1, Mux1/1, Delay4/1
  start/1 -> Vitis HLS/2
  Constant2/1 -> Vitis HLS/1

== system project5/Subsystem2 ==
  sel_in : Inport
  theta_in : Inport  Port=2
  start : Inport  Port=3
  Data_in2 : Inport  Port=4
  Constant2 : hdlBasic/Constant  const=0  gui_display_data_type=Boolean  arith_type=Boolean  n_bits=16  bin_pt=14  preci_type=Single  exp_width=8  frac_width=24  explicit_period=off  period=1  XmcBlockStatus=1  maskContainerNames=tabcontainer1  block_type=constant  block_config=sysgen:Constant_config
  Constant6 : hdlBasic/Constant  const=0  gui_display_data_type=Fixed-point  arith_type=Signed (2's comp)  n_bits=20  bin_pt=10  preci_type=Single  exp_width=8  frac_width=24  explicit_period=off  period=1  XmcBlockStatus=1  maskContainerNames=tabcontainer1  block_type=constant  block_config=sysgen:Constant_config
  Delay : hdlBasic/Delay  rst=off  en=on  latency=1  reg_retiming=off  XmcBlockStatus=1  maskContainerNames=group1  block_type=delay  block_config=sysgen:Delay_config
  Delay1 : hdlBasic/Delay  rst=off  en=on  latency=1  reg_retiming=off  XmcBlockStatus=1  maskContainerNames=group1  block_type=delay  block_config=sysgen:Delay_config
  Delay2 : hdlBasic/Delay  rst=off  en=off  latency=2  reg_retiming=off  XmcBlockStatus=1  maskContainerNames=group1  block_type=delay  block_config=sysgen:Delay_config
  Delay3 : hdlBasic/Delay  rst=off  en=off  latency=1  reg_retiming=off  XmcBlockStatus=1  maskContainerNames=group1  block_type=delay  block_config=sysgen:Delay_config
  Delay4 : hdlBasic/Delay  rst=off  en=off  latency=1  reg_retiming=off  XmcBlockStatus=1  maskContainerNames=group1  block_type=delay  block_config=sysgen:Delay_config
  Mux : hdlBasic/Mux  inputs=2  en=off  latency=1  precision=Full  arith_type=Unsigned  n_bits=16  bin_pt=14  quantization=Truncate  overflow=Wrap  XmcBlockStatus=1  maskContainerNames=tabcontainer1  block_type=mux  block_config=sysgen:Mux_config
  Mux1 : hdlBasic/Mux  inputs=2  en=off  latency=1  precision=Full  arith_type=Unsigned  n_bits=16  bin_pt=14  quantization=Truncate  overflow=Wrap  XmcBlockStatus=1  maskContainerNames=tabcontainer1  block_type=mux  block_config=sysgen:Mux_config
  Vitis HLS : hdlBasic/Vitis HLS  anytable='C:\ELEC522\jg122\Project5_sinandcos\sincos\solution1'  fast_sim=off  display_datatype=off  rate_propagation_method=Simulink system period  model_file_path=''  latency=1  block_type=vitis_hls
      settings: infoedit=This block allows including C,C++ and SystemC source files in System Generator for DSP designs.
  Ctrl_out : Outport
  theta_out : Outport  Port=2
  result_out : Outport  Port=3
  y_out : Outport  Port=4
  wires:
  Vitis HLS/4 -> Delay/1
  Vitis HLS/5 -> Delay/2
  Delay1/1 -> y_out/1
  Vitis HLS/7 -> Delay1/2
  Vitis HLS/6 -> Delay1/1
  sel_in/1 -> Delay4/1, Mux/1, Mux1/1
  Delay/1 -> result_out/1, Mux/2
  Constant6/1 -> Mux1/3
  Data_in2/1 -> Mux1/2, Mux/3
  Mux1/1 -> Vitis HLS/4
  Mux/1 -> Delay2/1
  theta_in/1 -> Vitis HLS/3, Delay3/1
  Delay3/1 -> theta_out/1
  Delay2/1 -> Vitis HLS/5
  Delay4/1 -> Ctrl_out/1
  start/1 -> Vitis HLS/2
  Constant2/1 -> Vitis HLS/1

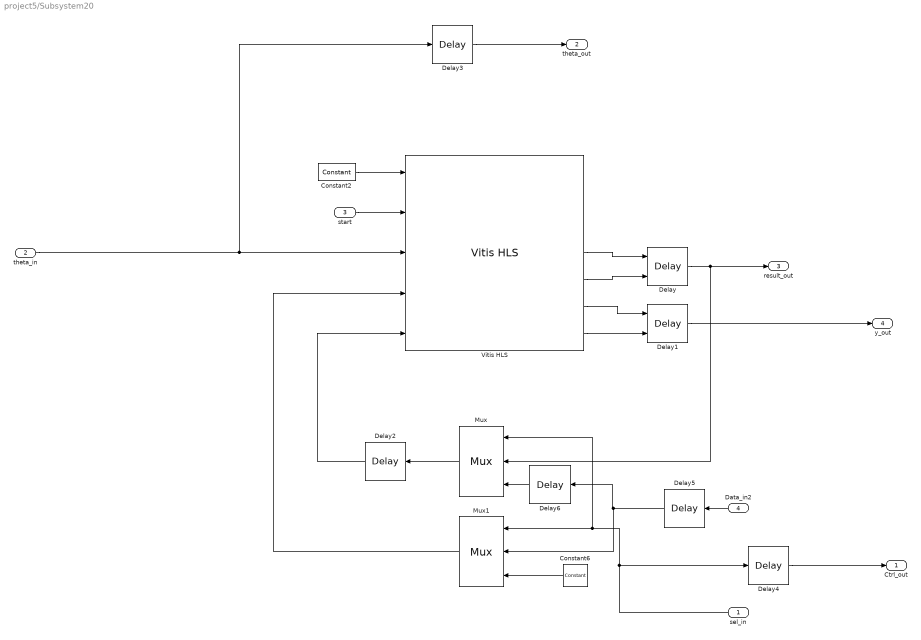
== system project5/Subsystem20 ==
  sel_in : Inport
  theta_in : Inport  Port=2
  start : Inport  Port=3
  Data_in2 : Inport  Port=4
  Constant2 : hdlBasic/Constant  const=0  gui_display_data_type=Boolean  arith_type=Boolean  n_bits=16  bin_pt=14  preci_type=Single  exp_width=8  frac_width=24  explicit_period=off  period=1  XmcBlockStatus=1  maskContainerNames=tabcontainer1  block_type=constant  block_config=sysgen:Constant_config
  Constant6 : hdlBasic/Constant  const=0  gui_display_data_type=Fixed-point  arith_type=Signed (2's comp)  n_bits=20  bin_pt=10  preci_type=Single  exp_width=8  frac_width=24  explicit_period=off  period=1  XmcBlockStatus=1  maskContainerNames=tabcontainer1  block_type=constant  block_config=sysgen:Constant_config
  Delay : hdlBasic/Delay  rst=off  en=on  latency=1  reg_retiming=off  XmcBlockStatus=1  maskContainerNames=group1  block_type=delay  block_config=sysgen:Delay_config
  Delay1 : hdlBasic/Delay  rst=off  en=on  latency=1  reg_retiming=off  XmcBlockStatus=1  maskContainerNames=group1  block_type=delay  block_config=sysgen:Delay_config
  Delay2 : hdlBasic/Delay  rst=off  en=off  latency=2  reg_retiming=off  XmcBlockStatus=1  maskContainerNames=group1  block_type=delay  block_config=sysgen:Delay_config
  Delay3 : hdlBasic/Delay  rst=off  en=off  latency=1  reg_retiming=off  XmcBlockStatus=1  maskContainerNames=group1  block_type=delay  block_config=sysgen:Delay_config
  Delay4 : hdlBasic/Delay  rst=off  en=off  latency=1  reg_retiming=off  XmcBlockStatus=1  maskContainerNames=group1  block_type=delay  block_config=sysgen:Delay_config
  Delay5 : hdlBasic/Delay  rst=off  en=off  latency=19  reg_retiming=off  XmcBlockStatus=1  maskContainerNames=group1  block_type=delay  block_config=sysgen:Delay_config
  Delay6 : hdlBasic/Delay  rst=off  en=off  latency=25  reg_retiming=off  XmcBlockStatus=1  maskContainerNames=group1  block_type=delay  block_config=sysgen:Delay_config
  Mux : hdlBasic/Mux  inputs=2  en=off  latency=1  precision=Full  arith_type=Unsigned  n_bits=16  bin_pt=14  quantization=Truncate  overflow=Wrap  XmcBlockStatus=1  maskContainerNames=tabcontainer1  block_type=mux  block_config=sysgen:Mux_config
  Mux1 : hdlBasic/Mux  inputs=2  en=off  latency=1  precision=Full  arith_type=Unsigned  n_bits=16  bin_pt=14  quantization=Truncate  overflow=Wrap  XmcBlockStatus=1  maskContainerNames=tabcontainer1  block_type=mux  block_config=sysgen:Mux_config
  Vitis HLS : hdlBasic/Vitis HLS  anytable='C:\ELEC522\jg122\Project5_sinandcos\sincos\solution1'  fast_sim=off  display_datatype=off  rate_propagation_method=Simulink system period  model_file_path=''  latency=1  block_type=vitis_hls
      settings: infoedit=This block allows including C,C++ and SystemC source files in System Generator for DSP designs.
  Ctrl_out : Outport
  theta_out : Outport  Port=2
  result_out : Outport  Port=3
  y_out : Outport  Port=4
  wires:
  Vitis HLS/4 -> Delay/1
  Vitis HLS/5 -> Delay/2
  Delay1/1 -> y_out/1
  Vitis HLS/7 -> Delay1/2
  Vitis HLS/6 -> Delay1/1
  Delay/1 -> result_out/1, Mux/2
  Constant6/1 -> Mux1/3
  Data_in2/1 -> Delay5/1
  Mux1/1 -> Vitis HLS/4
  Mux/1 -> Delay2/1
  theta_in/1 -> Vitis HLS/3, Delay3/1
  Delay3/1 -> theta_out/1
  Delay2/1 -> Vitis HLS/5
  Delay4/1 -> Ctrl_out/1
  Delay5/1 -> Mux1/2, Delay6/1
  Delay6/1 -> Mux/3
  sel_in/1 -> Mux/1, Mux1/1, Delay4/1
  start/1 -> Vitis HLS/2
  Constant2/1 -> Vitis HLS/1

== system project5/Subsystem21 ==
  Input_2 : Inport
  Input_1 : Inport  Port=2
  AddSub : hdlBasic/AddSub  mode=Addition  use_carryin=off  use_carryout=off  en=off  latency=0  precision=Full  arith_type=Unsigned  n_bits=16  bin_pt=14  quantization=Truncate  overflow=Wrap  use_behavioral_HDL=off  hw_selection=Fabric  pipelined=off  XmcBlockStatus=1  maskContainerNames=tabcontainer1  block_type=addsub  block_config=sysgen:Addsub_config
  AddSub1 : hdlBasic/AddSub  mode=Addition  use_carryin=off  use_carryout=off  en=off  latency=0  precision=Full  arith_type=Unsigned  n_bits=16  bin_pt=14  quantization=Truncate  overflow=Wrap  use_behavioral_HDL=off  hw_selection=Fabric  pipelined=off  XmcBlockStatus=1  maskContainerNames=tabcontainer1  block_type=addsub  block_config=sysgen:Addsub_config
  AddSub2 : hdlBasic/AddSub  mode=Addition  use_carryin=off  use_carryout=off  en=off  latency=0  precision=Full  arith_type=Unsigned  n_bits=16  bin_pt=14  quantization=Truncate  overflow=Wrap  use_behavioral_HDL=off  hw_selection=Fabric  pipelined=off  XmcBlockStatus=1  maskContainerNames=tabcontainer1  block_type=addsub  block_config=sysgen:Addsub_config
  Delay{,1..4} (5 alike) : hdlBasic/Delay  rst=off  en=off  latency=1  reg_retiming=off  XmcBlockStatus=1  maskContainerNames=group1  block_type=delay  block_config=sysgen:Delay_config
  Mult : hdlBasic/Mult  precision=User Defined  arith_type="Signed  (2's comp)"  n_bits=20  bin_pt=10  quantization=Truncate  overflow=Wrap  en=off  latency=0  use_behavioral_HDL=off  opt=Speed  use_embedded=on  optimum_pipeline=off  pipeline=on  use_rpm=on  placement_style=Triangular  XmcBlockStatus=1  maskContainerNames=group1  block_type=mult  block_config=sysgen:Mult_config
  Output_2 : Outport
  Result_out : Outport  Port=2
  Output_1 : Outport  Port=3
  wires:
  Input_1/1 -> Mult/1, Delay/1
  Input_2/1 -> Mult/2, Delay1/1
  Delay/1 -> Output_1/1
  Delay1/1 -> Output_2/1
  Delay2/1 -> Delay4/1, AddSub/1
  AddSub/1 -> AddSub1/2
  Mult/1 -> Delay2/1, AddSub/2
  Delay4/1 -> Delay3/1, AddSub1/1
  AddSub1/1 -> AddSub2/2
  AddSub2/1 -> Result_out/1
  Delay3/1 -> AddSub2/1

== system project5/Subsystem22 ==
  Input_2 : Inport
  Input_1 : Inport  Port=2
  AddSub : hdlBasic/AddSub  mode=Addition  use_carryin=off  use_carryout=off  en=off  latency=0  precision=Full  arith_type=Unsigned  n_bits=16  bin_pt=14  quantization=Truncate  overflow=Wrap  use_behavioral_HDL=off  hw_selection=Fabric  pipelined=off  XmcBlockStatus=1  maskContainerNames=tabcontainer1  block_type=addsub  block_config=sysgen:Addsub_config
  AddSub1 : hdlBasic/AddSub  mode=Addition  use_carryin=off  use_carryout=off  en=off  latency=0  precision=Full  arith_type=Unsigned  n_bits=16  bin_pt=14  quantization=Truncate  overflow=Wrap  use_behavioral_HDL=off  hw_selection=Fabric  pipelined=off  XmcBlockStatus=1  maskContainerNames=tabcontainer1  block_type=addsub  block_config=sysgen:Addsub_config
  AddSub3 : hdlBasic/AddSub  mode=Addition  use_carryin=off  use_carryout=off  en=off  latency=0  precision=Full  arith_type=Unsigned  n_bits=16  bin_pt=14  quantization=Truncate  overflow=Wrap  use_behavioral_HDL=off  hw_selection=Fabric  pipelined=off  XmcBlockStatus=1  maskContainerNames=tabcontainer1  block_type=addsub  block_config=sysgen:Addsub_config
  Delay{,1..2,4,6} (5 alike) : hdlBasic/Delay  rst=off  en=off  latency=1  reg_retiming=off  XmcBlockStatus=1  maskContainerNames=group1  block_type=delay  block_config=sysgen:Delay_config
  Mult : hdlBasic/Mult  precision=User Defined  arith_type="Signed  (2's comp)"  n_bits=20  bin_pt=10  quantization=Truncate  overflow=Wrap  en=off  latency=0  use_behavioral_HDL=off  opt=Speed  use_embedded=on  optimum_pipeline=off  pipeline=on  use_rpm=on  placement_style=Triangular  XmcBlockStatus=1  maskContainerNames=group1  block_type=mult  block_config=sysgen:Mult_config
  Output_2 : Outport
  Result_out : Outport  Port=2
  Output_1 : Outport  Port=3
  wires:
  Input_1/1 -> Mult/1, Delay/1
  Input_2/1 -> Mult/2, Delay1/1
  Delay/1 -> Output_1/1
  Delay1/1 -> Output_2/1
  Delay2/1 -> Delay4/1, AddSub/1
  AddSub/1 -> AddSub1/2
  Mult/1 -> Delay2/1, AddSub/2
  Delay4/1 -> Delay6/1, AddSub1/1
  AddSub1/1 -> AddSub3/2
  Delay6/1 -> AddSub3/1
  AddSub3/1 -> Result_out/1
